simulink model "R2RSystemModel"  (R2014a)
settings: Solver=ode45  StartTime=0.0  StopTime=60  RelTol=1e-3
undefined symbols (not defined in the file): K_L12_Force, K_PWM, L12_Offset_I, Mar, Ra_L12
settings Model: Creator=oberstare  LastModifiedBy=oberstare

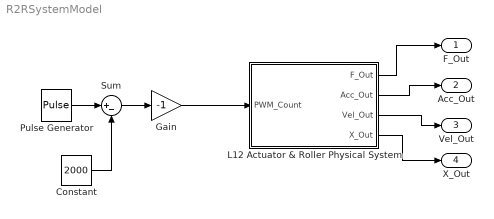
== system R2RSystemModel ==
  Constant : Constant  Value=2000
  Gain : Gain  Gain=-1
  L12 Actuator & Roller Physical System : Subsystem
  Pulse Generator : DiscretePulseGenerator  PulseType=Time based  Amplitude=4000  Period=20  PulseWidth=50  PhaseDelay=5
  Sum : Sum  Inputs=|+-
  F_Out : Outport
  Acc_Out : Outport  Port=2
  Vel_Out : Outport  Port=3
  X_Out : Outport  Port=4
  wires:
  L12 Actuator & Roller Physical System/1(F_Out) -> F_Out/1
  L12 Actuator & Roller Physical System/2(Acc_Out) -> Acc_Out/1
  L12 Actuator & Roller Physical System/3(Vel_Out) -> Vel_Out/1
  L12 Actuator & Roller Physical System/4(X_Out) -> X_Out/1
  Pulse Generator/1 -> Sum/1
  Constant/1 -> Sum/2
  Sum/1 -> Gain/1
  Gain/1 -> L12 Actuator & Roller Physical System/1(PWM_Count)

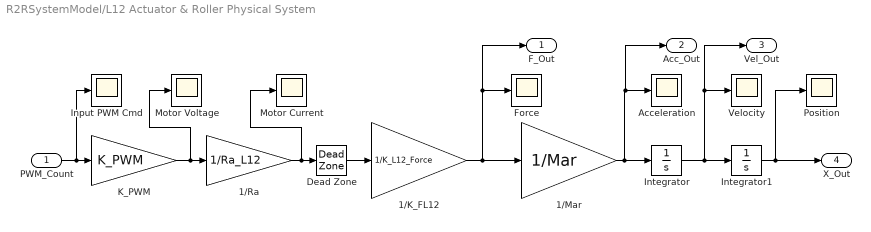
== system R2RSystemModel/L12 Actuator & Roller Physical System ==
  PWM_Count : Inport
  1/K_FL12 : Gain  Gain=1/K_L12_Force
  1/Mar : Gain  Gain=1/Mar
  1/Ra : Gain  Gain=1/Ra_L12
  Acceleration : Scope
      settings: SaveName=ScopeData4
  Dead Zone : DeadZone  LowerValue=-L12_Offset_I  UpperValue=L12_Offset_I  SaturateOnIntegerOverflow=on
  Force : Scope
      settings: TimeRange=12  YMin=-1.59375  YMax=2.40625
  Input PWM Cmd : Scope
      settings: AttributesFormatString=%<ShowName>
  Integrator : Integrator
  Integrator1 : Integrator
  K_PWM : Gain  Gain=K_PWM
  Motor Current : Scope
      settings: SaveName=ScopeData6
  Motor Voltage : Scope
      settings: SaveName=ScopeData5
  Position : Scope
      settings: SaveName=ScopeData3
  Velocity : Scope
      settings: SaveName=ScopeData2
  F_Out : Outport
  Acc_Out : Outport  Port=2
  Vel_Out : Outport  Port=3
  X_Out : Outport  Port=4
  wires:
  PWM_Count/1 -> Input PWM Cmd/1, K_PWM/1
  1/Mar/1 -> Acc_Out/1, Acceleration/1, Integrator/1
  Integrator1/1 -> X_Out/1, Position/1
  1/K_FL12/1 -> 1/Mar/1, F_Out/1, Force/1
  1/Ra/1 -> Dead Zone/1, Motor Current/1
  K_PWM/1 -> Motor Voltage/1, 1/Ra/1
  Integrator/1 -> Vel_Out/1, Velocity/1, Integrator1/1
  Dead Zone/1 -> 1/K_FL12/1
